simulink model "my_brake_actuator"  (R2024a)
settings: Solver=FixedStepDiscrete  StartTime=0.0  StopTime=10.0  FixedStep=0.005  RelTol=1e-3
model workspace (MATLAB code in the model file):
  | HBridgeCmd_LkupTbl = Simulink.LookupTable;
  | HBridgeCmd_LkupTbl.Table.DataType = 'int16';
  | HBridgeCmd_LkupTbl.Table.FieldName = 'Table';
  | HBridgeCmd_LkupTbl.Table.Value = int16( ...
  |   [-2048 -1843 -1638 -1434 -1229 -1024 -819 -614 -410 -205 0 205 410 614 ...
  |    819 1024 1229 1434 1638 1843 2048]);
  | HBridgeCmd_LkupTbl.BreakpointsSpecification = 'Explicit values';
  | HBridgeCmd_LkupTbl.SupportTunableSize = false;
  | HBridgeCmd_LkupTbl.Breakpoints.DataType = 'single';
  | HBridgeCmd_LkupTbl.Breakpoints.FieldName = 'BP1';
  | HBridgeCmd_LkupTbl.Breakpoints.Value = ...
  |   [-100 -90 -80 -70 -60 -50 -40 -30 -20 -10 0 10 20 30 40 50 60 70 80 90 ...
  |    100];
  | HBridgeCmd_LkupTbl.Breakpoints.TunableSizeName = 'N1';
  | HBridgeCmd_LkupTbl.StructTypeInfo.Name = 'MyStruct_Actuator';
  | HBridgeCmd_LkupTbl.StructTypeInfo.HeaderFileName = 'Rte_Type.h';
undefined symbols (not defined in the file or in its folder): TPSPercentBkpt, TPSPercentTbl
settings Model: Creator=The MathWorks, Inc.  LastModifiedBy=Mhamed
settings SolverCC: AlgebraicLoopSolver=TrustRegion  MaxZcPerStep=1
settings DataIOCC: SaveFormat=StructureWithTime  ReturnWorkspaceOutputs=off
settings OptimizationCC: DefaultParameterBehavior=Inlined  ReuseModelBlockBuffer=off  PassReuseOutputArgsAs=Individual arguments  ZeroExternalMemoryAtStartup=off  ZeroInternalMemoryAtStartup=off  EfficientTunableParamExpr=on
settings DebuggingCC: ParameterTunabilityLossMsg=error  UnconnectedInputMsg=warning  UnconnectedOutputMsg=warning  UnconnectedLineMsg=warning  ArithmeticOperatorsInVariantConditions=warning
settings ModelReferenceCC: EnableRefExpFcnMdlSchedulingChecks=on
settings SFSimCC: SimUseLocalCustomCode=off  MATLABDynamicMemAlloc=off  CustomCodeUndefinedFunction=UseInterfaceOnly
settings RTWCC: Description=AUTOSAR  SystemTargetFile=autosar.tlc  GenCodeOnly=on  TemplateMakefile=ert_default_tmf  GenerateReport=on  RTWUseLocalCustomCode=off  IncludeHyperlinkInReport=on  LaunchReport=on  DataTypeReplacement=CDataTypesFixedWidth  GenerateTraceInfo=on  GenerateTraceReport=on  GenerateTraceReportSl=on  GenerateTraceReportSf=on  GenerateTraceReportEml=on  GPUComputeCapability=3.5
settings CodeAppCC: ForceParamTrailComments=on  IgnoreCustomStorageClasses=off  OperatorAnnotations=on  SimulinkDataObjDesc=on  SFDataObjDesc=on  InsertBlockDesc=on
settings STFCustomTargetCC: MultiwordLength=256  ParMdlRefBuildCompliant=on  CompOptLevelCompliant=on  IncludeMdlTerminateFcn=off  CombineOutputUpdateFcns=on  SuppressErrorStatus=on  ERTCustomFileBanners=on  SupportNonFinite=off  SupportComplex=off  SupportContinuousTime=off  SupportNonInlinedSFcns=off  RemoveResetFunc=on  MATLABClassNameForMDSCustomization=Simulink.SoftwareTarget.ERTCustomization  CPPClassGenCompliant=on  AutosarCompliant=on  GRTInterface=off  LookupTableObjectStructAxisOrder=2,1,3,4,...  LUTObjectStructOrderEvenSpacing=Size,Table,Breakpoints  SystemTargetFile=autosar.tlc
settings ERTTargetCC: TargetLangStandard=C99 (ISO)  ConcurrentExecutionCompliant=off  IncludeMdlTerminateFcn=off  SuppressErrorStatus=on  SupportNonFinite=off  SupportComplex=off  ModelStepFunctionPrototypeControlCompliant=off  AutosarCompliant=on  LookupTableObjectStructAxisOrder=2,1,3,4,...  LUTObjectStructOrderEvenSpacing=Size,Table,Breakpoints  InlinedParameterPlacement=NonHierarchical  ERTCustomFileTemplate=example_file_process.tlc  BooleanTrueId=TRUE  BooleanFalseId=FALSE

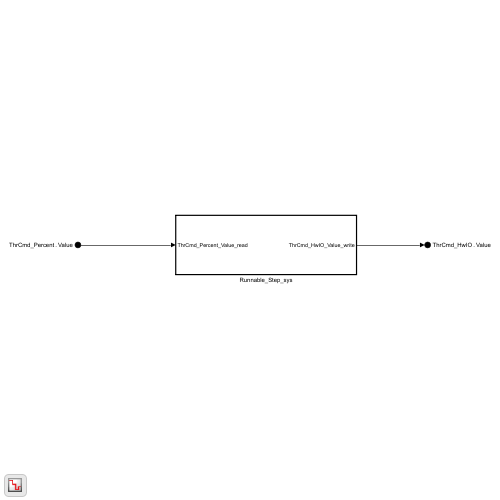
[thumbnail: Simulink's stored preview of the top-level diagram]
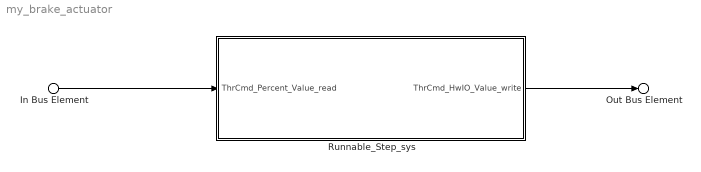
== system my_brake_actuator ==
  In Bus Element : Inport  PortName=ThrCmd_Percent  Element=Value
  Runnable_Step_sys : Subsystem  TreatAsAtomicUnit=on  SystemSampleTime=0.005
  Out Bus Element : Outport  PortName=ThrCmd_HwIO  Element=Value
  wires:
  In Bus Element/1 -> Runnable_Step_sys/1(ThrCmd_Percent_Value_read)
  Runnable_Step_sys/1(ThrCmd_HwIO_Value_write) -> Out Bus Element/1

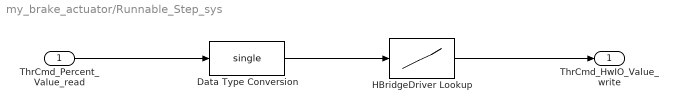
== system my_brake_actuator/Runnable_Step_sys ==
  ThrCmd_Percent_Value_read : Inport
  Data Type Conversion : DataTypeConversion  OutDataTypeStr=single  SaturateOnIntegerOverflow=off  RndMeth=Floor
  HBridgeDriver Lookup : Lookup_n-D  NumberOfTableDimensions=1  DataSpecification=Lookup table object  LookupTableObject=HBridgeCmd_LkupTbl  BreakpointsForDimension1=TPSPercentBkpt  BreakpointsForDimension1DataTypeStr=single  IndexSearchMethod=Linear search  Table=TPSPercentTbl  TableDataTypeStr=single  InterpMethod=Nearest  InternalRulePriority=Speed  OutDataTypeStr=Inherit: Inherit from 'Table data'  RndMeth=Simplest
  ThrCmd_HwIO_Value_write : Outport  VectorParamsAs1DForOutWhenUnconnected=off
  wires:
  ThrCmd_Percent_Value_read/1 -> Data Type Conversion/1
  HBridgeDriver Lookup/1 -> ThrCmd_HwIO_Value_write/1
  Data Type Conversion/1 -> HBridgeDriver Lookup/1
